simulink model "main_model_fd_v06_switchobservability"  (R2025a)
settings: Solver=ode3  StartTime=0.0  StopTime=1.5  FixedStep=1e-6  RelTol=1e-3
model workspace (MAT data in the model file):
  EP_ENERGY_INITIAL = 176
  EP_PBAT_SIGN = 1
  EP_PLOAD_SIGN = -1
  EP_POWER_ALPHA = 0.951229424501
  EP_POWER_BALANCE_ALPHA = 0.951229424501
  EP_POWER_CONFIRM_TIME = 0.01
  EP_POWER_FILTER_TAU = 0.002
  EP_PSOURCE_SIGN = 1
  EP_P_CHARGE_TRIP = 3000
  EP_P_CHARGE_WARN = 2500
  EP_P_DISCHARGE_TRIP = 3000
  EP_P_DISCHARGE_WARN = 2500
  EP_SOC_CHARGE_RELEASE = 88
  EP_SOC_CHARGE_STOP = 90
  EP_SOC_DISCHARGE_RELEASE = 12
  EP_SOC_DISCHARGE_STOP = 10
  EP_SOC_WARN_HIGH = 85
  EP_SOC_WARN_LOW = 15
  EP_TS = 0.0001
  FD_CBUS = 0.0022
  FD_CBUS_ESR = 0.001
  FD_CURRENT_QUANT_STEP = 1e-06
  FD_DUTY_BIAS = 0
  FD_DUTY_STUCK_ENABLE = 0
  FD_DUTY_STUCK_VALUE = 0.5
  FD_FAULT_END_TIME = 1000000000
  FD_FAULT_ID = 0
  FD_FAULT_TIME = 0.8
  FD_IBAT_BIAS = 0
  FD_IBAT_NOISE_STD = 0
  FD_IBAT_TRIP = 20
  FD_IL_BIAS = 0
  FD_IL_NOISE_STD = 0
  FD_IL_TRIP = 15
  FD_IREF_LEVEL = 10
  FD_IREF_OVERRIDE_ENABLE = 0
  FD_LOAD_STEP_A = 0
  FD_LOAD_STEP_TIME = 0.5
  FD_L_MAIN = 0.015
  FD_MODE_COMMAND = 2
  FD_MODE_OVERRIDE_ENABLE = 0
  FD_PROTECTION_ARM_TIME = 0.15
  FD_PROTECTION_MODE = 2
  FD_RBAT = 0.5
  FD_S1_FAULT_PULSE_WIDTH = 0
  FD_S1_OPEN = 0
  FD_S2_FAULT_PULSE_WIDTH = 0
  FD_S2_OPEN = 0
  FD_SENSOR_TS = 5e-05
  FD_SWITCH_FAULT_PERIOD = 0.0005
  FD_TRIP_DELAY_STEPS = 20000
  FD_TS = 1e-06
  FD_VBAT_BIAS = 0
  FD_VBAT_NOISE_STD = 0
  FD_VBAT_QUANT_STEP = 1e-06
  FD_VBUS_BIAS = 0
  FD_VBUS_HI = 430
  FD_VBUS_LO = 360
  FD_VBUS_NOISE_STD = 0
  FD_VBUS_QUANT_STEP = 1e-06
  I_charge_max = 10
  I_discharge_cmd = 10
  RandomSeed = 240727
  SOCInit = 20
  Var10 = 0
  Var11 = 0
  Var6 = 0
  Var7 = 0
  Var8 = 0
  Var9 = 0
undefined symbols (not defined in the file): DiscIntNeverNeededParam, dspblkCoreblockFVToolHelper, gcbh, Ion, Lithium
libraries: hdlsllib x17, spsSeriesRLCBranchLib x6, spsCurrentMeasurementLib x3, simulink x2, spsIGBTDiodeLib x2, eeGeneralControl x2, slpidlib x2, spsVoltageMeasurementLib x2, spsBatteryLib x1, spsControlledVoltageSourceLib x1, spsControlledCurrentSourceLib x1, spsPWMGeneratorDCDCLib x1
(part 2 of 2)

== stateflow chart main_model_fd_v06_switchobservability/Mode_Manager ==
  settings: updateMethod=DISCRETE  sampleTime=1e-3
  state Standby
    entry:
    Iref_target = 0;
    gate_enable = false;
    mode_id = 0;
    transition_flag = false;
    reset_pi = true;
    during:
    Iref_target = 0;
    gate_enable = false;
    mode_id = 0;
    transition_flag = false;
    reset_pi = false;
  state Precharge
    entry:
    Iref_target = 0;
    gate_enable = false;
    mode_id = 1;
    transition_flag = true;
    reset_pi = true;
    during:
    Iref_target = 0;
    gate_enable = false;
    mode_id = 1;
    transition_flag = true;
    reset_pi = false;
  state Charge
    entry,during:
    Iref_target = FD_IREF_OVERRIDE_ENABLE*FD_IREF_LEVEL + (1-FD_IREF_OVERRIDE_ENABLE)*Iref_bus_raw;
    gate_enable = true;
    mode_id = 2;
    transition_flag = false;
    reset_pi = false;
  state Discharge
    entry,during:
    Iref_target = FD_IREF_OVERRIDE_ENABLE*(-FD_IREF_LEVEL) + (1-FD_IREF_OVERRIDE_ENABLE)*Iref_bus_raw;
    gate_enable = true;
    mode_id = 3;
    transition_flag = false;
    reset_pi = false;
  state Transition
    entry,during:
    Iref_target = 0;
    gate_enable = true;
    mode_id = 4;
    transition_flag = true;
    reset_pi = false
  state Fault_lockout
    entry,during:
    Iref_target = 0;
    gate_enable = false;
    mode_id = 5;
    transition_flag = false;
    reset_pi = true;
  (default) -> Standby
  Fault_lockout -> Standby : [fault_reset && ~trip]
  Standby -> Fault_lockout [order 1] : [trip]
  Transition -> Standby [order 3] : [duration(abs(I_L_avg)<I_zero)>=0.005 && mode_cmd==0]
  Standby -> Precharge [order 2] : [(mode_cmd==1 && charge_allowed) ||(mode_cmd==2 && discharge_allowed)]
  Precharge -> Standby [order 4] : [(mode_cmd==0) || (mode_cmd==1 && ~charge_allowed) ||(mode_cmd==2 && ~discharge_allowed)]
  Transition -> Precharge [order 2] : [duration(abs(I_L_avg)<I_zero)>=0.005 && mode_cmd~=0]
  Precharge -> Fault_lockout [order 1] : [trip]
  Precharge -> Charge [order 2] : [after(5,msec) && mode_cmd==1 && charge_allowed]
  Precharge -> Discharge [order 3] : [after(5,msec) && mode_cmd==2 && discharge_allowed]
  Discharge -> Transition [order 2] : [mode_cmd~=2 || ~discharge_allowed]
  Discharge -> Fault_lockout [order 1] : [trip]
  Charge -> Fault_lockout [order 1] : [trip]
  Charge -> Transition [order 2] : [mode_cmd~=1 || ~charge_allowed]
  Transition -> Fault_lockout [order 1] : [trip]
  data: mode_cmd input double; I_L_avg input double; charge_allowed input boolean; fault_reset input boolean; trip input boolean; discharge_allowed input boolean; Iref_target output double; gate_enable output boolean; mode_id output double; transition_flag output boolean; reset_pi output boolean; I_zero constant double =0.5; Iref_bus_raw input double; FD_IREF_OVERRIDE_ENABLE parameter double; FD_IREF_LEVEL parameter double

== stateflow chart main_model_fd_v06_switchobservability/mod_cmd ==
  state STANDBY
    entry,during:
    mod_cmd = 0;
  state Charge_request
    entry,during:
    mod_cmd = 1;
  state Discharge_request1
    entry,during:
    mod_cmd = 2;
  (default) -> STANDBY
  STANDBY -> Charge_request [order 1] : [duration(V_bus>= V_charge_on) >= T_enter]
  Charge_request -> STANDBY : [duration(V_bus <= V_charge_off) >= T_exit]
  Discharge_request1 -> STANDBY : [duration(V_bus >= V_discharge_off) >= T_exit]
  STANDBY -> Discharge_request1 [order 2] : [duration(V_bus <= V_discharge_on) >= T_enter]
  data: V_charge_off constant double =399.5; V_discharge_on constant double =398; V_discharge_off constant double =400.5; T_enter constant double =0.01; T_exit constant double =0.02; V_bus input; mod_cmd output; V_charge_on constant double =402
